simulink model "ROSACE_VA_control_simu"  (Simulink 7.8)
settings: Solver=FixedStepDiscrete  StartTime=0.0  StopTime=100  FixedStep=dt  RelTol=1e-3
values from neighbouring files (symbols this model uses):
  A_de = [0  1; -625  -42.5]    [simu_data.mat]    (also in simu_data_dyn.m = [0 1;-omega^2 -2*xi*omega])
  A_dx = -0.75    [simu_data.mat]    (also in simu_data_dyn.m = [-0.75])
  alpha_0 = -0.05    [simu_data.mat]    (also in simu_data_const.m)
  Az_q = [0  -0.766000101841; 1  1.73490320589]    [simu_data.mat]    (also in simu_data_dyn.m = [0 1;-G_q.den{1}(end:-1:2)]')
  Az_Va = [0  -0.956543675476; 1  1.95557839805]    [simu_data.mat]    (also in simu_data_dyn.m = [0 1;-G_Va.den{1}(end:-1:2)]')
  Az_Vz = [0  -0.956543675476; 1  1.95557839805]    [simu_data.mat]    (also in simu_data_dyn.m = [0 1;-G_Vz.den{1}(end:-1:2)]')
  B_de = [0 625]    [simu_data.mat]    (also in simu_data_dyn.m = [0 omega^2]')
  B_dx = 0.75    [simu_data.mat]    (also in simu_data_dyn.m = [0.75]')
  Bz_q = [0.0148576489814 0.016239246974]    [simu_data.mat]    (also in simu_data_dyn.m = [G_q.num{1}(end:-1:2)]')
  Bz_Va = [0.000479064865372 0.000486212556349]    [simu_data.mat]    (also in simu_data_dyn.m = [G_Va.num{1}(end:-1:2)]')
  Bz_Vz = [0.000479064865372 0.000486212556349]    [simu_data.mat]    (also in simu_data_dyn.m = [G_Vz.num{1}(end:-1:2)]')
  C_de = [1 0]    [simu_data.mat]    (also in simu_data_dyn.m)
  C_dx = 26350    [simu_data.mat]    (also in simu_data_dyn.m = [26350])
  cbar = 4.29    [simu_data.mat]    (also in simu_data_const.m)
  CD_0 = 0.016    [simu_data.mat]    (also in simu_data_const.m)
  CD_alpha = 2.5    [simu_data.mat]    (also in simu_data_const.m)
  CD_deltae = 0.05    [simu_data.mat]    (also in simu_data_const.m)
  CI_de = [0.0120096156525 0]    [simu_data.mat]    (also in simu_data_dyn.m = [delta_e_eq 0])
  CI_dx = 1.58686607949    [simu_data.mat]    (also in simu_data_dyn.m = [delta_x_eq])
  CI_FD = [229.919332201 6.09103276514 0 0.0264858476817 10000]    [simu_data.mat]    (also in simu_data_dyn.m = [u0 w0 q0 theta0 h0])
  CIz_q = [0 0]    [simu_data.mat]    (also in simu_data_dyn.m)
  CIz_Va = [-219.89486044 230]    [simu_data.mat]    (also in simu_data_dyn.m = [1+G_Va.den{1}(2)-G_Va.num{1}(2) 1]*Va_eq)
  CIz_Vz = [0 0]    [simu_data.mat]    (also in simu_data_dyn.m)
  CL_alpha = 5.5    [simu_data.mat]    (also in simu_data_const.m)
  CL_deltae = 0.193    [simu_data.mat]    (also in simu_data_const.m)
  Cm_0 = 0.04    [simu_data.mat]    (also in simu_data_const.m)
  Cm_alpha = -0.83    [simu_data.mat]    (also in simu_data_const.m)
  Cm_deltae = -1.5    [simu_data.mat]    (also in simu_data_const.m)
  Cm_q = -30    [simu_data.mat]    (also in simu_data_const.m)
  Cz_q = [0 1]    [simu_data.mat]    (also in simu_data_dyn.m)
  Cz_Va = [0 1]    [simu_data.mat]    (also in simu_data_dyn.m)
  Cz_Vz = [0 1]    [simu_data.mat]    (also in simu_data_dyn.m)
  D_de = 0    [simu_data.mat]    (also in simu_data_dyn.m = [0])
  D_dx = 0    [simu_data.mat]    (also in simu_data_dyn.m = [0])
  delta_x_eq = 1.58686607949    [simu_data.mat]    (also in simu_data_const.m)
  dt_dx = 0.005    [allrates.mat]    (also in simu_data.mat; simu_data_const.m)
  Dz_q = 0    [simu_data.mat]    (also in simu_data_dyn.m = [0])
  Dz_Va = 0    [simu_data.mat]    (also in simu_data_dyn.m = [0])
  Dz_Vz = 0    [simu_data.mat]    (also in simu_data_dyn.m = [0])
  g0 = 9.80665    [simu_data.mat]    (also in simu_data_const.m)
  I_y = 3781272    [simu_data.mat]    (also in simu_data_const.m)
  K1_intVa = 0.0498026106644    [simu_data.mat]    (also in simu_data_const.m)
  K1_q = 21.6923833763    [simu_data.mat]    (also in simu_data_const.m)
  K1_Va = -0.486813084356    [simu_data.mat]    (also in simu_data_const.m)
  K1_Vz = -0.0776030954954    [simu_data.mat]    (also in simu_data_const.m)
  mass = 57837.5    [simu_data.mat]    (also in simu_data_const.m)
  rho0 = 1.225    [simu_data.mat]    (also in simu_data_const.m)
  Rs = 287.05    [simu_data.mat]    (also in simu_data_const.m)
  S = 122.6    [simu_data.mat]    (also in simu_data_const.m)
  T0_0 = 288.15    [simu_data.mat]    (also in simu_data_const.m)
  T0_h = -0.0065    [simu_data.mat]    (also in simu_data_const.m)
  Ts_f_q = 0.01    [allrates.mat]    (also in simu_data.mat; simu_data_const.m)
  Ts_f_Va = 0.01    [allrates.mat]    (also in simu_data.mat; simu_data_const.m)
  Ts_f_Vz = 0.01    [allrates.mat]    (also in simu_data.mat; simu_data_const.m)
  Ts_K1 = 0.02    [allrates.mat]    (also in simu_data.mat; simu_data_const.m)
  Va_eq = 230    [simu_data.mat]    (also in simu_data_const.m)
undefined symbols (not defined in the file or in its folder): DiscIntNeverNeededParam, magnitude
settings Model: Creator=David  LastModifiedBy=tloquen  ExtModeAutoUpdateStatusClock=off
settings DataIOCC: LimitDataPoints=off
settings DebuggingCC: SaveWithParameterizedLinksMsg=none  MultiTaskDSMMsg=warning  MultiTaskCondExecSysMsg=none
settings HardwareCC: TargetHWDeviceType=32-bit Generic
settings SFSimCC: SimParseCustomCode=off
settings RTWCC: IncludeERTFirstTime=on
settings CodeAppCC: CustomSymbolStrType=$N$R$M_T
settings GRTTargetCC: TargetFcnLib=ansi_tfl_tmw.mat

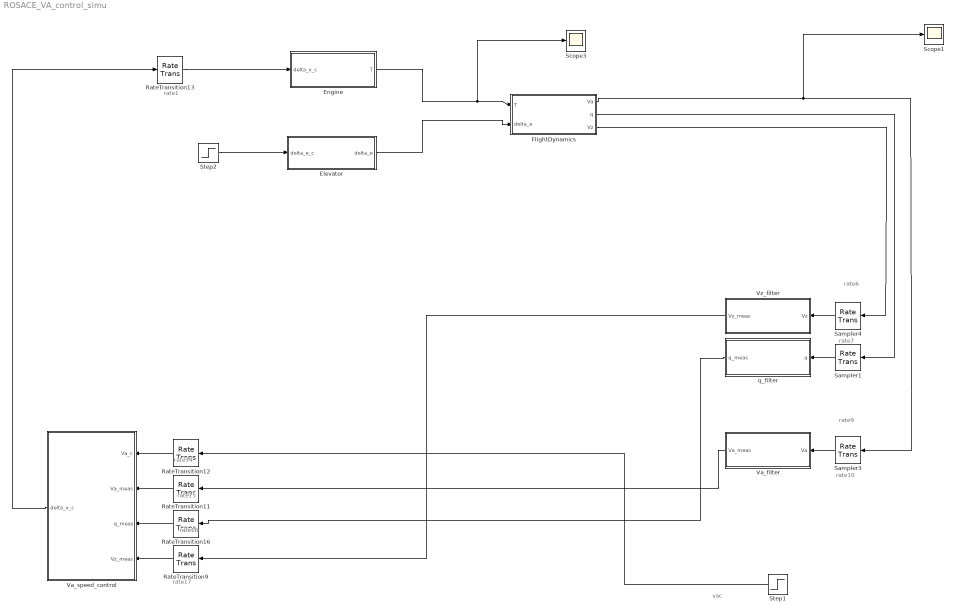
== system ROSACE_VA_control_simu ==
  note: rate1
  note: rate6
  note: rate7
  note: rate9
  note: rate10
  note: rate14
  note: rate15
  note: rate16
  note: rate17
  note: vac
  Elevator : Subsystem
  Engine : Subsystem
  FlightDynamics : Subsystem
  RateTransition{9,11..12,16} (4 alike) : RateTransition  OutPortSampleTime=Ts_K1
  RateTransition13 : RateTransition  X0=delta_x_eq  OutPortSampleTime=dt_dx
  Sampler1 : RateTransition  OutPortSampleTime=Ts_f_q
  Sampler3 : RateTransition  X0=Va_eq  OutPortSampleTime=Ts_f_Va
      settings: AttributesFormatString=%<Name>
  Sampler4 : RateTransition  OutPortSampleTime=Ts_f_Vz
  Scope1 : Scope
      settings: SaveName=ScopeData2
  Scope3 : Scope
      settings: SaveName=ScopeData6
  Step1 : Step  After=235  SampleTime=0  VectorParams1D=off
  Step2 : Step  After=14e-3  SampleTime=0
  Va_filter : Subsystem
  Va_speed_control : Subsystem
  "Vz_filter " : Subsystem
  q_filter : Subsystem
  wires:
  Step1/1 -> RateTransition12/1
  FlightDynamics/1(Va) -> Sampler3/1, Scope1/1
  FlightDynamics/2(q) -> Sampler1/1
  FlightDynamics/3(Vz) -> Sampler4/1
  Engine/1(T) -> FlightDynamics/1(T), Scope3/1
  Elevator/1(delta_e) -> FlightDynamics/2(delta_e)
  Va_filter/1(Va_meas) -> RateTransition11/1
  q_filter/1(q_meas) -> RateTransition16/1
  RateTransition11/1 -> Va_speed_control/2(Va_meas)
  RateTransition12/1 -> Va_speed_control/1(Va_c)
  Va_speed_control/1(delta_x_c) -> RateTransition13/1
  RateTransition13/1 -> Engine/1(delta_x_c)
  RateTransition16/1 -> Va_speed_control/3(q_meas)
  "Vz_filter "/1(Vz_meas) -> RateTransition9/1
  RateTransition9/1 -> Va_speed_control/4(Vz_meas)
  Sampler4/1 -> "Vz_filter "/1(Vz)
  Sampler1/1 -> q_filter/1(q)
  Sampler3/1 -> Va_filter/1(Va)
  Step2/1 -> Elevator/1(delta_e_c)

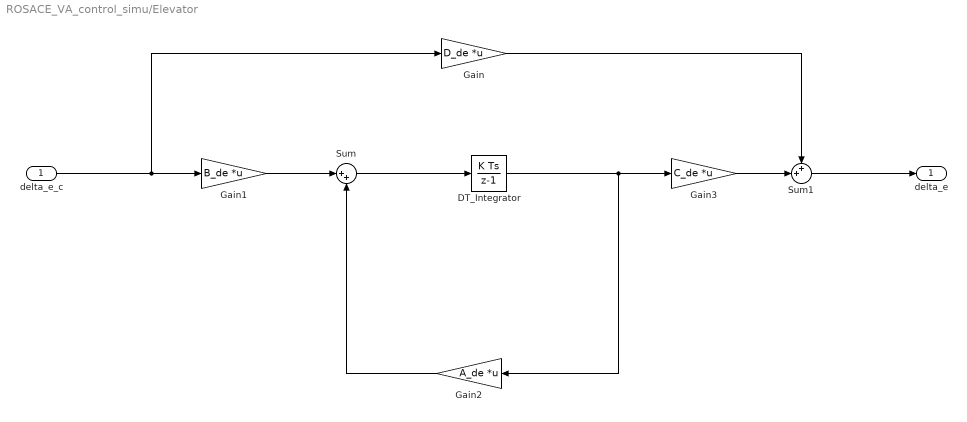
== system ROSACE_VA_control_simu/Elevator ==
  delta_e_c : Inport
  DT_Integrator : DiscreteIntegrator  InitialCondition=CI_de  SampleTime=dt_dx  ICPrevOutput=DiscIntNeverNeededParam  ICPrevScaledInput=DiscIntNeverNeededParam
  Gain : Gain  Gain=D_de  Multiplication=Matrix(K*u)  OutDataTypeStr=Inherit: Same as input  ParamDataTypeStr=Inherit: Same as input
  Gain1 : Gain  Gain=B_de  Multiplication=Matrix(K*u)  OutDataTypeStr=Inherit: Same as input  ParamDataTypeStr=Inherit: Same as input
  Gain2 : Gain  Gain=A_de  Multiplication=Matrix(K*u)  OutDataTypeStr=Inherit: Same as input  ParamDataTypeStr=Inherit: Same as input
  Gain3 : Gain  Gain=C_de  Multiplication=Matrix(K*u)  OutDataTypeStr=Inherit: Same as input  ParamDataTypeStr=Inherit: Same as input
  Sum : Sum  Inputs=|++  OutDataTypeStr=Inherit: Same as first input
  Sum1 : Sum  Inputs=++|  OutDataTypeStr=Inherit: Same as first input
  delta_e : Outport
  wires:
  delta_e_c/1 -> Gain/1, Gain1/1
  Sum1/1 -> delta_e/1
  Sum/1 -> DT_Integrator/1
  Gain/1 -> Sum1/1
  Gain1/1 -> Sum/1
  Gain2/1 -> Sum/2
  Gain3/1 -> Sum1/2
  DT_Integrator/1 -> Gain2/1, Gain3/1

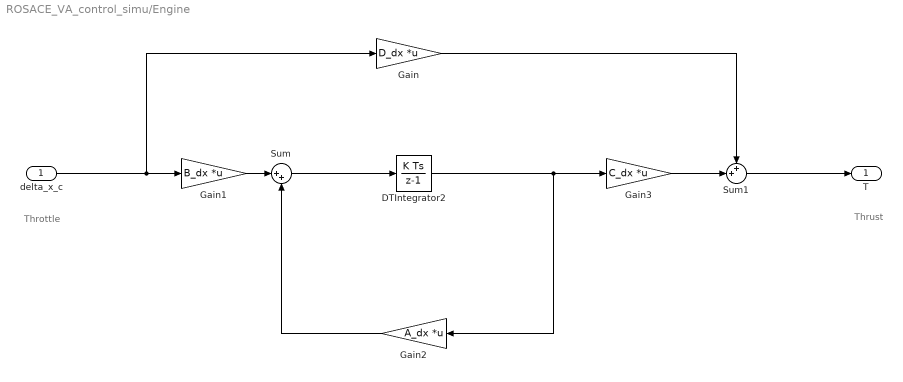
== system ROSACE_VA_control_simu/Engine ==
  note: Throttle
  note: Thrust
  delta_x_c : Inport
  DTIntegrator2 : DiscreteIntegrator  InitialCondition=CI_dx  SampleTime=dt_dx  ICPrevOutput=DiscIntNeverNeededParam  ICPrevScaledInput=DiscIntNeverNeededParam
  Gain : Gain  Gain=D_dx  Multiplication=Matrix(K*u)  OutDataTypeStr=Inherit: Same as input  ParamDataTypeStr=Inherit: Same as input
  Gain1 : Gain  Gain=B_dx  Multiplication=Matrix(K*u)  OutDataTypeStr=Inherit: Same as input  ParamDataTypeStr=Inherit: Same as input
  Gain2 : Gain  Gain=A_dx  Multiplication=Matrix(K*u)  OutDataTypeStr=Inherit: Same as input  ParamDataTypeStr=Inherit: Same as input
  Gain3 : Gain  Gain=C_dx  Multiplication=Matrix(K*u)  OutDataTypeStr=Inherit: Same as input  ParamDataTypeStr=Inherit: Same as input
  Sum : Sum  Inputs=|++  OutDataTypeStr=Inherit: Same as first input
  Sum1 : Sum  Inputs=++|  OutDataTypeStr=Inherit: Same as first input
  T : Outport
  wires:
  delta_x_c/1 -> Gain/1, Gain1/1
  Sum1/1 -> T/1
  DTIntegrator2/1 -> Gain2/1, Gain3/1
  Sum/1 -> DTIntegrator2/1
  Gain/1 -> Sum1/1
  Gain1/1 -> Sum/1
  Gain2/1 -> Sum/2
  Gain3/1 -> Sum1/2

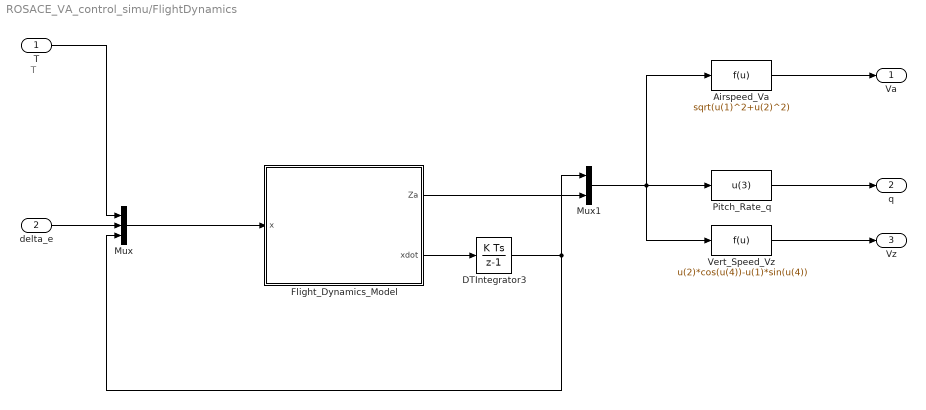
== system ROSACE_VA_control_simu/FlightDynamics ==
  note: T
  T : Inport
  delta_e : Inport  Port=2
  "Airspeed_Va  " : Fcn  Expr=sqrt(u(1)^2+u(2)^2)
  DTIntegrator3 : DiscreteIntegrator  InitialCondition=CI_FD  SampleTime=dt_dx  ICPrevOutput=DiscIntNeverNeededParam  ICPrevScaledInput=DiscIntNeverNeededParam
  Flight_Dynamics_Model : Subsystem
  Mux : Mux  Inputs=3
  Mux1 : Mux  Inputs=2
  "Pitch_Rate_q " : Fcn  Expr=u(3)
  Vert_Speed_Vz : Fcn  Expr=u(2)*cos(u(4))-u(1)*sin(u(4))
  Va : Outport
  q : Outport  Port=2
  Vz : Outport  Port=3
  wires:
  delta_e/1 -> Mux/2
  DTIntegrator3/1 -> Mux/3, Mux1/1
  T/1 -> Mux/1
  Mux/1 -> Flight_Dynamics_Model/1(x)
  Flight_Dynamics_Model/2(xdot) -> DTIntegrator3/1
  Vert_Speed_Vz/1 -> Vz/1
  "Pitch_Rate_q "/1 -> q/1
  "Airspeed_Va  "/1 -> Va/1
  Flight_Dynamics_Model/1(Za) -> Mux1/2
  Mux1/1 -> "Pitch_Rate_q "/1, "Airspeed_Va  "/1, Vert_Speed_Vz/1

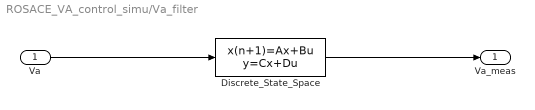
== system ROSACE_VA_control_simu/Va_filter ==
  Va : Inport
  Discrete_State_Space : DiscreteStateSpace  A=Az_Va  B=Bz_Va  C=Cz_Va  D=Dz_Va  X0=CIz_Va  SampleTime=Ts_f_Va
  Va_meas : Outport
  wires:
  Discrete_State_Space/1 -> Va_meas/1
  Va/1 -> Discrete_State_Space/1

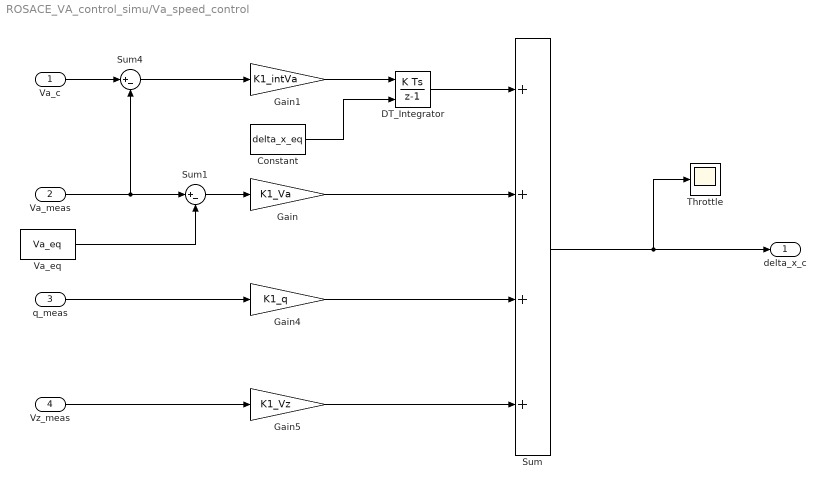
== system ROSACE_VA_control_simu/Va_speed_control ==
  Va_c : Inport
  Va_meas : Inport  Port=2
  q_meas : Inport  Port=3
  Vz_meas : Inport  Port=4
  Constant : Constant  Value=delta_x_eq  SampleTime=Ts_K1
  DT_Integrator : DiscreteIntegrator  InitialConditionSource=external  SampleTime=Ts_K1  ICPrevOutput=DiscIntNeverNeededParam  ICPrevScaledInput=DiscIntNeverNeededParam
  Gain : Gain  Gain=K1_Va  OutDataTypeStr=Inherit: Same as input  ParamDataTypeStr=Inherit: Same as input
  Gain1 : Gain  Gain=K1_intVa  OutDataTypeStr=Inherit: Same as input  ParamDataTypeStr=Inherit: Same as input
  Gain4 : Gain  Gain=K1_q  OutDataTypeStr=Inherit: Same as input  ParamDataTypeStr=Inherit: Same as input
  Gain5 : Gain  Gain=K1_Vz  OutDataTypeStr=Inherit: Same as input  ParamDataTypeStr=Inherit: Same as input
  Sum : Sum  Inputs=++++  SampleTime=Ts_K1  OutDataTypeStr=Inherit: Same as first input
  Sum1 : Sum  Inputs=|+-  SampleTime=Ts_K1  OutDataTypeStr=Inherit: Same as first input
  Sum4 : Sum  Inputs=|+-  SampleTime=Ts_K1  OutDataTypeStr=Inherit: Same as first input
  Throttle : Scope
      settings: YMin=10094  YMax=10100.5  SaveName=ScopeData5  DataFormat=Array
  Va_eq : Constant  Value=Va_eq  SampleTime=Ts_K1
  delta_x_c : Outport
  wires:
  Va_meas/1 -> Sum1/1, Sum4/2
  Sum1/1 -> Gain/1
  Gain/1 -> Sum/2
  Va_c/1 -> Sum4/1
  Gain1/1 -> DT_Integrator/1
  q_meas/1 -> Gain4/1
  Vz_meas/1 -> Gain5/1
  Gain4/1 -> Sum/3
  Gain5/1 -> Sum/4
  Sum/1 -> Throttle/1, delta_x_c/1
  Constant/1 -> DT_Integrator/2
  Va_eq/1 -> Sum1/2
  Sum4/1 -> Gain1/1
  DT_Integrator/1 -> Sum/1

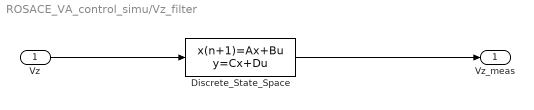
== system ROSACE_VA_control_simu/Vz_filter  ==
  Vz : Inport
  Discrete_State_Space : DiscreteStateSpace  A=Az_Vz  B=Bz_Vz  C=Cz_Vz  D=Dz_Vz  X0=CIz_Vz  SampleTime=Ts_f_Vz
  Vz_meas : Outport
  wires:
  Discrete_State_Space/1 -> Vz_meas/1
  Vz/1 -> Discrete_State_Space/1

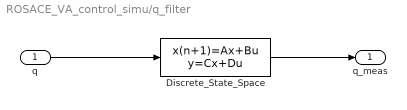
== system ROSACE_VA_control_simu/q_filter ==
  q : Inport
  Discrete_State_Space : DiscreteStateSpace  A=Az_q  B=Bz_q  C=Cz_q  D=Dz_q  X0=CIz_q  SampleTime=Ts_f_q
  q_meas : Outport
  wires:
  Discrete_State_Space/1 -> q_meas/1
  q/1 -> Discrete_State_Space/1

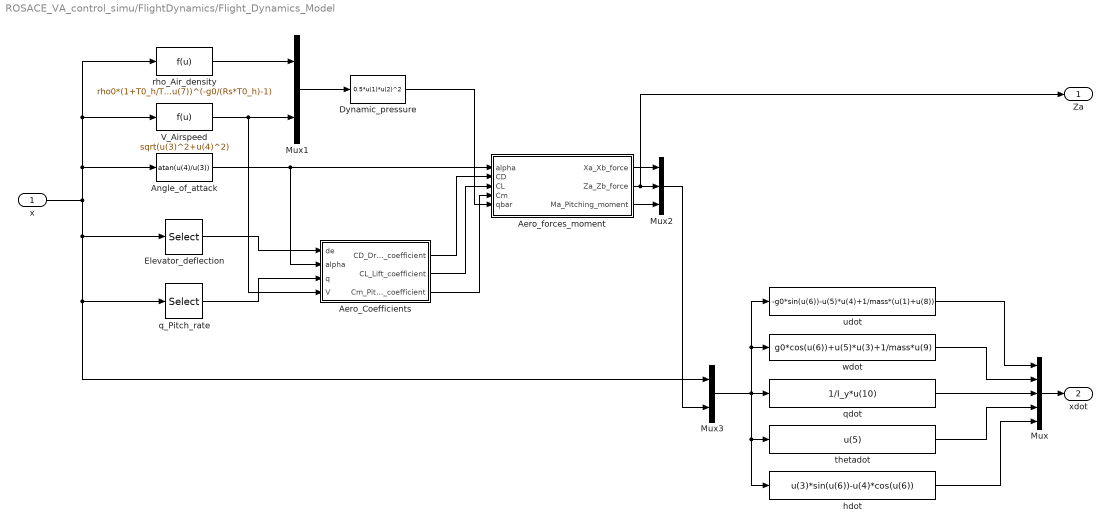
== system ROSACE_VA_control_simu/FlightDynamics/Flight_Dynamics_Model ==
  x : Inport
  Aero_Coefficients : Subsystem
  Aero_forces_moment : Subsystem
  Angle_of_attack : Fcn  Expr=atan(u(4)/u(3))
  Dynamic_pressure : Fcn  Expr=0.5*u(1)*u(2)^2
  Elevator_deflection : Selector  InputPortWidth=7  IndexOptions=Index vector (dialog)  Indices=[2]  OutputSizes=1
  Mux : Mux  Inputs=5
  Mux1 : Mux  Inputs=2
  Mux2 : Mux  Inputs=3
  Mux3 : Mux  Inputs=2
  V_Airspeed : Fcn  Expr=sqrt(u(3)^2+u(4)^2)
  hdot : Fcn  Expr=u(3)*sin(u(6))-u(4)*cos(u(6))
  q_Pitch_rate : Selector  InputPortWidth=7  IndexOptions=Index vector (dialog)  Indices=[5]  OutputSizes=1
  qdot : Fcn  Expr=1/I_y*u(10)
  rho_Air_density : Fcn  Expr=rho0*(1+T0_h/T0_0*u(7))^(-g0/(Rs*T0_h)-1)
  thetadot : Fcn  Expr=u(5)
  udot : Fcn  Expr=-g0*sin(u(6))-u(5)*u(4)+1/mass*(u(1)+u(8))
  wdot : Fcn  Expr=g0*cos(u(6))+u(5)*u(3)+1/mass*u(9)
  Za : Outport
  xdot : Outport  Port=2
  wires:
  udot/1 -> Mux/1
  wdot/1 -> Mux/2
  qdot/1 -> Mux/3
  thetadot/1 -> Mux/4
  hdot/1 -> Mux/5
  Mux/1 -> xdot/1
  x/1 -> Elevator_deflection/1, q_Pitch_rate/1, Mux3/1, rho_Air_density/1, V_Airspeed/1, Angle_of_attack/1
  rho_Air_density/1 -> Mux1/1
  V_Airspeed/1 -> Mux1/2, Aero_Coefficients/4(V)
  Mux1/1 -> Dynamic_pressure/1
  Angle_of_attack/1 -> Aero_forces_moment/1(alpha), Aero_Coefficients/2(alpha)
  Dynamic_pressure/1 -> Aero_forces_moment/5(qbar)
  Aero_forces_moment/1("Xa_Xb_force ") -> Mux2/1
  Aero_forces_moment/2(Za_Zb_force) -> Za/1, Mux2/2
  Aero_forces_moment/3(Ma_Pitching_moment) -> Mux2/3
  Mux2/1 -> Mux3/2
  Mux3/1 -> wdot/1, udot/1, qdot/1, thetadot/1, hdot/1
  Elevator_deflection/1 -> Aero_Coefficients/1(de)
  q_Pitch_rate/1 -> Aero_Coefficients/3(q)
  Aero_Coefficients/1(CD_Drag_coefficient) -> Aero_forces_moment/2(CD)
  Aero_Coefficients/2(CL_Lift_coefficient) -> Aero_forces_moment/3(CL)
  Aero_Coefficients/3(Cm_Pitching_coefficient) -> Aero_forces_moment/4(Cm)

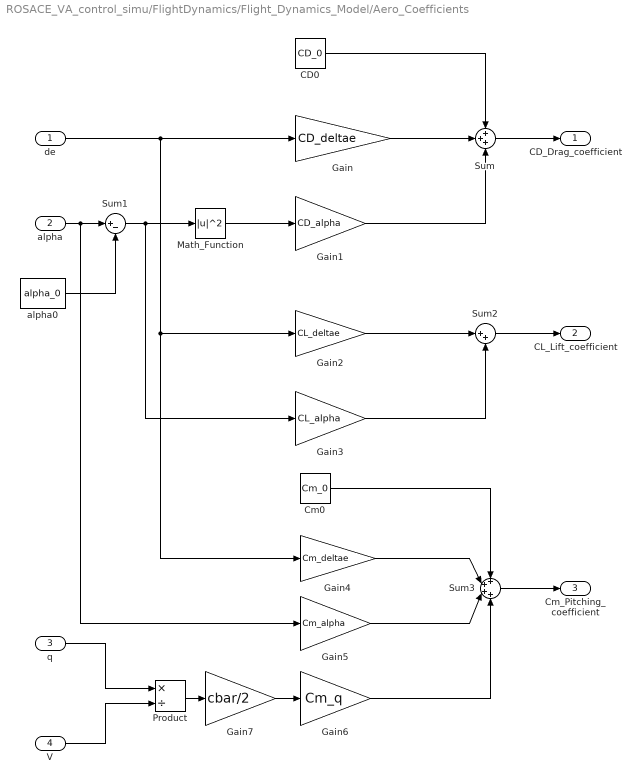
== system ROSACE_VA_control_simu/FlightDynamics/Flight_Dynamics_Model/Aero_Coefficients ==
  de : Inport
  alpha : Inport  Port=2
  q : Inport  Port=3
  V : Inport  Port=4
  CD0 : Constant  Value=CD_0  SampleTime=-1
  Cm0 : Constant  Value=Cm_0  SampleTime=-1
  Gain : Gain  Gain=CD_deltae  OutDataTypeStr=Inherit: Same as input  ParamDataTypeStr=Inherit: Same as input
  Gain1 : Gain  Gain=CD_alpha  OutDataTypeStr=Inherit: Same as input  ParamDataTypeStr=Inherit: Same as input
  Gain2 : Gain  Gain=CL_deltae  OutDataTypeStr=Inherit: Same as input  ParamDataTypeStr=Inherit: Same as input
  Gain3 : Gain  Gain=CL_alpha  OutDataTypeStr=Inherit: Same as input  ParamDataTypeStr=Inherit: Same as input
  Gain4 : Gain  Gain=Cm_deltae  OutDataTypeStr=Inherit: Same as input  ParamDataTypeStr=Inherit: Same as input
  Gain5 : Gain  Gain=Cm_alpha  OutDataTypeStr=Inherit: Same as input  ParamDataTypeStr=Inherit: Same as input
  Gain6 : Gain  Gain=Cm_q  OutDataTypeStr=Inherit: Same as input  ParamDataTypeStr=Inherit: Same as input
  Gain7 : Gain  Gain=cbar/2  OutDataTypeStr=Inherit: Same as input  ParamDataTypeStr=Inherit: Same as input
  Math_Function : Math  Operator=magnitude^2  SaturateOnIntegerOverflow=on
  Product : Product  Inputs=*/  RndMeth=Zero  OutDataTypeStr=Inherit: Same as first input
  Sum : Sum  Inputs=+++  OutDataTypeStr=Inherit: Same as first input
  Sum1 : Sum  Inputs=|+-  OutDataTypeStr=Inherit: Same as first input
  Sum2 : Sum  Inputs=|++  OutDataTypeStr=Inherit: Same as first input
  Sum3 : Sum  Inputs=++++  OutDataTypeStr=Inherit: Same as first input
  alpha0 : Constant  Value=alpha_0  SampleTime=-1
  CD_Drag_coefficient : Outport
  CL_Lift_coefficient : Outport  Port=2
  Cm_Pitching_coefficient : Outport  Port=3
  wires:
  de/1 -> Gain/1, Gain2/1, Gain4/1
  CD0/1 -> Sum/1
  Gain/1 -> Sum/2
  Gain1/1 -> Sum/3
  Sum/1 -> CD_Drag_coefficient/1
  alpha/1 -> Sum1/1, Gain5/1
  alpha0/1 -> Sum1/2
  Sum1/1 -> Math_Function/1, Gain3/1
  Math_Function/1 -> Gain1/1
  Gain3/1 -> Sum2/2
  Sum2/1 -> CL_Lift_coefficient/1
  Gain2/1 -> Sum2/1
  Cm0/1 -> Sum3/1
  Gain4/1 -> Sum3/2
  Gain5/1 -> Sum3/3
  Sum3/1 -> Cm_Pitching_coefficient/1
  Gain6/1 -> Sum3/4
  q/1 -> Product/1
  V/1 -> Product/2
  Product/1 -> Gain7/1
  Gain7/1 -> Gain6/1

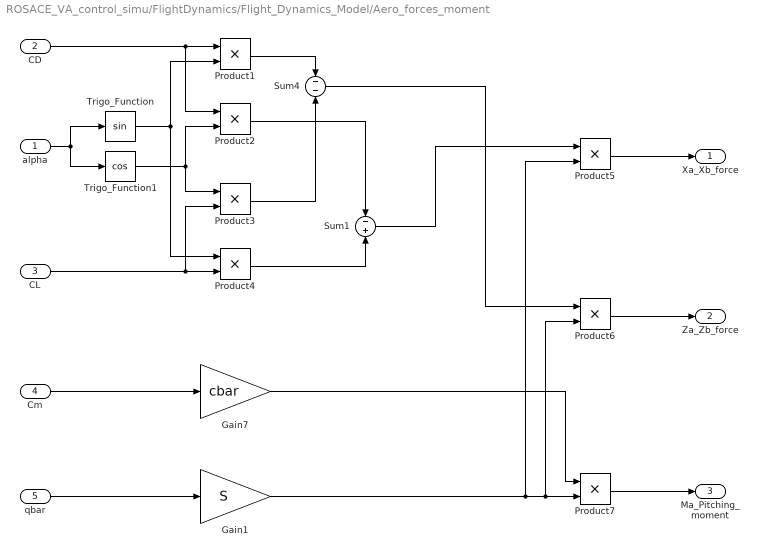
== system ROSACE_VA_control_simu/FlightDynamics/Flight_Dynamics_Model/Aero_forces_moment ==
  alpha : Inport
  CD : Inport  Port=2
  CL : Inport  Port=3
  Cm : Inport  Port=4
  qbar : Inport  Port=5
  Gain1 : Gain  Gain=S  OutDataTypeStr=Inherit: Same as input  ParamDataTypeStr=Inherit: Same as input
  Gain7 : Gain  Gain=cbar  OutDataTypeStr=Inherit: Same as input  ParamDataTypeStr=Inherit: Same as input
  Product{1..7} (7 alike) : Product  RndMeth=Zero  OutDataTypeStr=Inherit: Same as first input
  Sum1 : Sum  Inputs=-+  OutDataTypeStr=Inherit: Same as first input
  Sum4 : Sum  Inputs=--  OutDataTypeStr=Inherit: Same as first input
  Trigo_Function : Trigonometry
  Trigo_Function1 : Trigonometry  Operator=cos
  "Xa_Xb_force " : Outport
  Za_Zb_force : Outport  Port=2
  Ma_Pitching_moment : Outport  Port=3
  wires:
  Product5/1 -> "Xa_Xb_force "/1
  Product6/1 -> Za_Zb_force/1
  Product7/1 -> Ma_Pitching_moment/1
  alpha/1 -> Trigo_Function/1, Trigo_Function1/1
  CD/1 -> Product1/1, Product2/1
  Trigo_Function/1 -> Product1/2, Product4/1
  Trigo_Function1/1 -> Product2/2, Product3/1
  CL/1 -> Product4/2, Product3/2
  Product4/1 -> Sum1/2
  Product2/1 -> Sum1/1
  Product1/1 -> Sum4/1
  Product3/1 -> Sum4/2
  Sum4/1 -> Product6/1
  Cm/1 -> Gain7/1
  Gain7/1 -> Product7/1
  Sum1/1 -> Product5/1
  qbar/1 -> Gain1/1
  Gain1/1 -> Product7/2, Product6/2, Product5/2
